simulink model "COSTEP_Auto"  (R2024b)
settings: Solver=FixedStepAuto  StartTime=0.0  StopTime=25  FixedStep=1/3600  RelTol=1e-3
model workspace (MAT data in the model file):
  AD : Simulink.Parameter (value not decoded)
  AG : Simulink.Parameter (value not decoded)
  AH : Simulink.Parameter (value not decoded)
  AV : Simulink.Parameter (value not decoded)
  AVP : Simulink.Parameter (value not decoded)
  BCHL : Simulink.Parameter (value not decoded)
  BCHV : Simulink.Parameter (value not decoded)
  BD : Simulink.Parameter (value not decoded)
  BG : Simulink.Parameter (value not decoded)
  BH : Simulink.Parameter (value not decoded)
  BVP : Simulink.Parameter (value not decoded)
  CD : Simulink.Parameter (value not decoded)
  CG : Simulink.Parameter (value not decoded)
  CH : Simulink.Parameter (value not decoded)
  CVP : Simulink.Parameter (value not decoded)
  ISV : Simulink.Parameter (value not decoded)
  XMW : Simulink.Parameter (value not decoded)
  XNS : Simulink.Parameter (value not decoded)
  XNS2 : Simulink.Parameter (value not decoded)
  XNS3 : Simulink.Parameter (value not decoded)
  XNSE : Simulink.Parameter (value not decoded)
values from neighbouring files (symbols this model uses):
  DD = SimData{4,1}{1,2}    [Auto_run_COSTEP.m]    (also in Run_COSTEP.m)
  G = SimData{2,1}(j,2)    [Auto_run_COSTEP.m]    (also in G.mat = [4243534565 7854912354 3456432354 1731738903 4346024432 5784; Run_COSTEP.m)
  IDV = SimData{3,1}(1:20,j)    [Auto_run_COSTEP.m]    (also in IDV.mat = [0 0 0 0 0 0 0 0 0 0 0 0 ... (812 elements, 28x29)]; Run_COSTEP.m = SimData{3,1}(1:28,j))
symbols that are objects in the model workspace (value not decoded): AD, AG, AH, AV, AVP, BD, BG, BH, BVP, CD, CG, CH, CVP, XMW, XNS, XNS2, XNS3, XNSE
undefined symbols (not defined in the file or in its folder): magnitude, msgbox, SETPT, XMEAS, XMV
libraries: mylib x304, dspindex x31
(part 5 of 13)

== system COSTEP_Auto/Process Measurements/Product analysis/Subsystem ==
  <XST(I;13)> : Inport
  Bus Selector : BusSelector  OutputSignals=XMNS(37),XMNS(38),XMNS(39),XMNS(40),XMNS(41)
  Process Noise I=37-{1..4,41} (5 alike) : mylib/Process Noise I=37-41  SystemSampleTime=-1  VariantActivationTime=update diagram  AllowFlexibleInterface=on  Latency=0  AutoFrameSizeCalculation=off
  Subsystem : Subsystem
  XMEAS(37) : Outport  VectorParamsAs1DForOutWhenUnconnected=off
  XMEAS(38) : Outport  Port=2  VectorParamsAs1DForOutWhenUnconnected=off
  XMEAS(39) : Outport  Port=3  VectorParamsAs1DForOutWhenUnconnected=off
  XMEAS(40) : Outport  Port=4  VectorParamsAs1DForOutWhenUnconnected=off
  XMEAS(41) : Outport  Port=5  VectorParamsAs1DForOutWhenUnconnected=off
  wires:
  Process Noise I=37-41/1 -> XMEAS(37)/1
  Bus Selector/1 -> Process Noise I=37-41/2  "<XMNS(37)>"
  Process Noise I=37-1/1 -> XMEAS(38)/1
  Bus Selector/2 -> Process Noise I=37-1/2  "<XMNS(38)>"
  Process Noise I=37-2/1 -> XMEAS(39)/1
  Bus Selector/3 -> Process Noise I=37-2/2  "<XMNS(39)>"
  Process Noise I=37-3/1 -> XMEAS(40)/1
  Bus Selector/4 -> Process Noise I=37-3/2  "<XMNS(40)>"
  Process Noise I=37-4/1 -> XMEAS(41)/1
  Bus Selector/5 -> Process Noise I=37-4/2  "<XMNS(41)>"
  <XST(I;13)>/1 -> Subsystem/1(XST)
  Subsystem/1("XCMP(37) ") -> Process Noise I=37-41/1
  Subsystem/2("XCMP(38) ") -> Process Noise I=37-1/1
  Subsystem/3("XCMP(39) ") -> Process Noise I=37-2/1
  Subsystem/4("XCMP(40) ") -> Process Noise I=37-3/1
  Subsystem/5("XCMP(41) ") -> Process Noise I=37-4/1
  [XMNS3] -> Bus Selector/1

== system COSTEP_Auto/Process Measurements/Purge gas analysis/Subsystem ==
  <XST(I;10)> : Inport
  Bus Selector : BusSelector  OutputSignals=XMNS(29),XMNS(30),XMNS(31),XMNS(32),XMNS(33),XMNS(34),XMNS(35),XMNS(36)
  Process Noise I=23-{1..7,36} (8 alike) : mylib/Process Noise I=23-36  SystemSampleTime=-1  VariantActivationTime=update diagram  AllowFlexibleInterface=on  Latency=0  AutoFrameSizeCalculation=off
  Subsystem : Subsystem
  XMEAS(29) : Outport  VectorParamsAs1DForOutWhenUnconnected=off
  XMEAS(30) : Outport  Port=2  VectorParamsAs1DForOutWhenUnconnected=off
  XMEAS(31) : Outport  Port=3  VectorParamsAs1DForOutWhenUnconnected=off
  XMEAS(32) : Outport  Port=4  VectorParamsAs1DForOutWhenUnconnected=off
  XMEAS(33) : Outport  Port=5  VectorParamsAs1DForOutWhenUnconnected=off
  XMEAS(34) : Outport  Port=6  VectorParamsAs1DForOutWhenUnconnected=off
  XMEAS(35) : Outport  Port=7  VectorParamsAs1DForOutWhenUnconnected=off
  XMEAS(36) : Outport  Port=8  VectorParamsAs1DForOutWhenUnconnected=off
  wires:
  Process Noise I=23-36/1 -> XMEAS(29)/1
  Process Noise I=23-1/1 -> XMEAS(30)/1
  Bus Selector/2 -> Process Noise I=23-1/2  "<XMNS(30)>"
  Process Noise I=23-2/1 -> XMEAS(31)/1
  Process Noise I=23-3/1 -> XMEAS(32)/1
  Process Noise I=23-4/1 -> XMEAS(33)/1
  Process Noise I=23-5/1 -> XMEAS(34)/1
  Process Noise I=23-6/1 -> XMEAS(35)/1
  Process Noise I=23-7/1 -> XMEAS(36)/1
  Bus Selector/7 -> Process Noise I=23-6/2  "<XMNS(35)>"
  Bus Selector/8 -> Process Noise I=23-7/2  "<XMNS(36)>"
  Bus Selector/6 -> Process Noise I=23-5/2  "<XMNS(34)>"
  Bus Selector/5 -> Process Noise I=23-4/2  "<XMNS(33)>"
  Bus Selector/4 -> Process Noise I=23-3/2  "<XMNS(32)>"
  Bus Selector/3 -> Process Noise I=23-2/2  "<XMNS(31)>"
  Bus Selector/1 -> Process Noise I=23-36/2  "<XMNS(29)>"
  <XST(I;10)>/1 -> Subsystem/1(XST)
  Subsystem/1("XCMP(29) ") -> Process Noise I=23-36/1
  Subsystem/2("XCMP(30) ") -> Process Noise I=23-1/1
  Subsystem/3("XCMP(31) ") -> Process Noise I=23-2/1
  Subsystem/4("XCMP(32) ") -> Process Noise I=23-3/1
  Subsystem/5("XCMP(33) ") -> Process Noise I=23-4/1
  Subsystem/6("XCMP(34) ") -> Process Noise I=23-5/1
  Subsystem/7("XCMP(35) ") -> Process Noise I=23-6/1
  Subsystem/8("XCMP(36) ") -> Process Noise I=23-7/1
  [XMNS2] -> Bus Selector/1

== system COSTEP_Auto/Process Measurements/Reactor feed analysis/Subsystem ==
  <XST(I;6) = XST(I;7)> : Inport
  Bus Selector : BusSelector  OutputSignals=XMNS(23),XMNS(24),XMNS(25),XMNS(26),XMNS(27),XMNS(28)
  Process Noise I=23-{1..5,36} (6 alike) : mylib/Process Noise I=23-36  SystemSampleTime=-1  VariantActivationTime=update diagram  AllowFlexibleInterface=on  Latency=0  AutoFrameSizeCalculation=off
  Subsystem : Subsystem
  XMEAS(23) : Outport  VectorParamsAs1DForOutWhenUnconnected=off
  XMEAS(24) : Outport  Port=2  VectorParamsAs1DForOutWhenUnconnected=off
  XMEAS(25) : Outport  Port=3  VectorParamsAs1DForOutWhenUnconnected=off
  XMEAS(26) : Outport  Port=4  VectorParamsAs1DForOutWhenUnconnected=off
  XMEAS(27) : Outport  Port=5  VectorParamsAs1DForOutWhenUnconnected=off
  XMEAS(28) : Outport  Port=6  VectorParamsAs1DForOutWhenUnconnected=off
  wires:
  Process Noise I=23-36/1 -> XMEAS(23)/1
  Bus Selector/1 -> Process Noise I=23-36/2  "<XMNS(23)>"
  Process Noise I=23-1/1 -> XMEAS(24)/1
  Process Noise I=23-2/1 -> XMEAS(25)/1
  Process Noise I=23-3/1 -> XMEAS(26)/1
  Process Noise I=23-4/1 -> XMEAS(27)/1
  Process Noise I=23-5/1 -> XMEAS(28)/1
  Bus Selector/2 -> Process Noise I=23-1/2  "<XMNS(24)>"
  Bus Selector/3 -> Process Noise I=23-2/2  "<XMNS(25)>"
  Bus Selector/4 -> Process Noise I=23-3/2  "<XMNS(26)>"
  Bus Selector/6 -> Process Noise I=23-5/2  "<XMNS(28)>"
  <XST(I;6) = XST(I;7)>/1 -> Subsystem/1(XST)
  Subsystem/1(XCMP(23)1) -> Process Noise I=23-36/1
  Subsystem/2(XCMP(24)1) -> Process Noise I=23-1/1
  Subsystem/3(XCMP(25)1) -> Process Noise I=23-2/1
  Subsystem/4(XCMP(26)1) -> Process Noise I=23-3/1
  Subsystem/5(XCMP(27)1) -> Process Noise I=23-4/1
  Subsystem/6(XCMP(28)1) -> Process Noise I=23-5/1
  [XMNS2] -> Bus Selector/1
  Bus Selector/5 -> Process Noise I=23-4/2  "<XMNS(27)>"

== system COSTEP_Auto/Process Measurements/Subsystem3/Reactor Feed  ==
  " " : Constant  Value=35.3145
  "  " : Constant  Value=0.359
  Add : Sum
  Bus Selector : BusSelector  OutputSignals=signal1.FTM(6) = FTM(7)
  Bus Selector1 : BusSelector  OutputSignals=XMNS(6)
  Product1 : Product  Inputs=**/
  "XMEAS(6) " : Outport  VectorParamsAs1DForOutWhenUnconnected=off
  wires:
  " "/1 -> Product1/3
  "  "/1 -> Product1/2
  [PropertiesStream6] -> Bus Selector/1
  Bus Selector/1 -> Product1/1  "<FTM(6) = FTM(7)>"
  Product1/1 -> Add/1
  Add/1 -> "XMEAS(6) "/1  "XMEAS(6)"
  Bus Selector1/1 -> Add/2  "<XMNS(6)>"
  [XMNS] -> Bus Selector1/1

== system COSTEP_Auto/Process Measurements/Subsystem3/Reactor Level ==
  " " : Sum  Inputs=+-
  "    " : Constant  Value=84.6
  "      " : Constant  Value=666.7
  "       " : Constant  Value=100
  Add : Sum
  Bus Selector1 : BusSelector  OutputSignals=XMNS(8)
  XMEAS(8) : Product  Inputs=*/*
  "XMEAS(8) " : Outport  VectorParamsAs1DForOutWhenUnconnected=off
  wires:
  " "/1 -> XMEAS(8)/1
  "       "/1 -> XMEAS(8)/3
  "    "/1 -> " "/2
  [VLR] -> " "/1
  "      "/1 -> XMEAS(8)/2
  XMEAS(8)/1 -> Add/1
  Add/1 -> "XMEAS(8) "/1  "XMEAS(8)"
  Bus Selector1/1 -> Add/2  "<XMNS(8)>"
  [XMNS] -> Bus Selector1/1

== system COSTEP_Auto/Process Measurements/Subsystem3/Reactor Pressure ==
  " " : Sum  Inputs=+-
  "    " : Constant  Value=760
  "       " : Constant  Value=101.325
  Add : Sum
  Bus Selector1 : BusSelector  OutputSignals=XMNS(7)
  XMEAS(7) : Product  Inputs=*/*
  "XMEAS(7) " : Outport  VectorParamsAs1DForOutWhenUnconnected=off
  wires:
  " "/1 -> XMEAS(7)/1
  "       "/1 -> XMEAS(7)/3
  "    "/1 -> XMEAS(7)/2, " "/2
  [PTR] -> " "/1
  XMEAS(7)/1 -> Add/1
  Add/1 -> "XMEAS(7) "/1  "XMEAS(7)"
  Bus Selector1/1 -> Add/2  "<XMNS(7)>"
  [XMNS] -> Bus Selector1/1

== system COSTEP_Auto/Process Measurements/Subsystem3/Reactor Temperature ==
  Add : Sum
  Bus Selector1 : BusSelector  OutputSignals=XMNS(9)
  "XMEAS(9) " : Outport  VectorParamsAs1DForOutWhenUnconnected=off
  wires:
  [TCR] -> Add/1
  Add/1 -> "XMEAS(9) "/1  "XMEAS(9)"
  Bus Selector1/1 -> Add/2  "<XMNS(9)>"
  [XMNS] -> Bus Selector1/1

== system COSTEP_Auto/Process Measurements/Subsystem4/Purge Rate ==
  " " : Constant  Value=35.3145
  "  " : Constant  Value=0.359
  Add : Sum
  Bus Selector : BusSelector  OutputSignals=signal1.FTM(10)
  Bus Selector1 : BusSelector  OutputSignals=XMNS(10)
  Product1 : Product  Inputs=**/
  "XMEAS(10) " : Outport  VectorParamsAs1DForOutWhenUnconnected=off
  wires:
  " "/1 -> Product1/3
  Bus Selector/1 -> Product1/1  "<FTM(10)>"
  "  "/1 -> Product1/2
  [PropertiesStream10] -> Bus Selector/1
  Product1/1 -> Add/1
  Add/1 -> "XMEAS(10) "/1  "XMEAS(10)"
  Bus Selector1/1 -> Add/2  "<XMNS(10)>"
  [XMNS] -> Bus Selector1/1

== system COSTEP_Auto/Process Measurements/Subsystem4/Separator Level ==
  " " : Sum  Inputs=+-
  "    " : Constant  Value=27.5
  "      " : Constant  Value=290
  "       " : Constant  Value=100
  Add : Sum
  Bus Selector1 : BusSelector  OutputSignals=XMNS(12)
  XMEAS(12) : Product  Inputs=*/*
  "XMEAS(12) " : Outport  VectorParamsAs1DForOutWhenUnconnected=off
  wires:
  " "/1 -> XMEAS(12)/1
  "       "/1 -> XMEAS(12)/3
  "    "/1 -> " "/2
  [VLS] -> " "/1
  "      "/1 -> XMEAS(12)/2
  XMEAS(12)/1 -> Add/1
  Add/1 -> "XMEAS(12) "/1  "XMEAS(12)"
  [XMNS] -> Bus Selector1/1
  Bus Selector1/1 -> Add/2  "<XMNS(12)>"

== system COSTEP_Auto/Process Measurements/Subsystem4/Separator Pressure ==
  "       1" : Constant  Value=101.325
  "    1" : Constant  Value=760
  " 1" : Sum  Inputs=+-
  Add : Sum
  Bus Selector1 : BusSelector  OutputSignals=XMNS(13)
  XMEAS(13) : Product  Inputs=*/*
  "XMEAS(13) " : Outport  VectorParamsAs1DForOutWhenUnconnected=off
  wires:
  "       1"/1 -> XMEAS(13)/3
  "    1"/1 -> XMEAS(13)/2, " 1"/2
  " 1"/1 -> XMEAS(13)/1
  [PTS] -> " 1"/1
  XMEAS(13)/1 -> Add/1
  Add/1 -> "XMEAS(13) "/1  "XMEAS(13)"
  [XMNS] -> Bus Selector1/1
  Bus Selector1/1 -> Add/2  "<XMNS(13)>"

== system COSTEP_Auto/Process Measurements/Subsystem4/Separator Temperature ==
  Add : Sum
  Bus Selector1 : BusSelector  OutputSignals=XMNS(11)
  "XMEAS(11) " : Outport  VectorParamsAs1DForOutWhenUnconnected=off
  wires:
  [TCS] -> Add/1
  Add/1 -> "XMEAS(11) "/1  "XMEAS(11)"
  [XMNS] -> Bus Selector1/1
  Bus Selector1/1 -> Add/2  "<XMNS(11)>"

== system COSTEP_Auto/Process Measurements/Subsystem4/Separator Underflow ==
  "       " : Constant  Value=35.3145
  Add : Sum
  Bus Selector : BusSelector  OutputSignals=signal1.FTM(11)
  Bus Selector1 : BusSelector  OutputSignals=XMNS(14)
  XMEAS(14) : Product  Inputs=*//
  "XMEAS(14) " : Outport  VectorParamsAs1DForOutWhenUnconnected=off
  wires:
  "       "/1 -> XMEAS(14)/3
  [DLS] -> XMEAS(14)/2
  [PropertiesStream11] -> Bus Selector/1
  Bus Selector/1 -> XMEAS(14)/1  "<FTM(11)>"
  XMEAS(14)/1 -> Add/1
  Add/1 -> "XMEAS(14) "/1  "XMEAS(14)"
  [XMNS] -> Bus Selector1/1
  Bus Selector1/1 -> Add/2  "<XMNS(14)>"

== system COSTEP_Auto/Process Measurements/Subsystem5/Stripper Level ==
  " " : Sum  Inputs=+-
  "    " : Constant  Value=78.25
  "       " : Constant  Value=100
  Add : Sum
  Bus Selector1 : BusSelector  OutputSignals=XMNS(15)
  VTC Total Volume of Stripper ft³ : Constant  Value=156.5
  XMEAS(15) : Product  Inputs=*/*
  "XMEAS(15) " : Outport  VectorParamsAs1DForOutWhenUnconnected=off
  wires:
  " "/1 -> XMEAS(15)/1
  "       "/1 -> XMEAS(15)/3
  "    "/1 -> " "/2
  [VLC] -> " "/1
  VTC Total Volume of Stripper ft³/1 -> XMEAS(15)/2
  XMEAS(15)/1 -> Add/1
  Add/1 -> "XMEAS(15) "/1  "XMEAS(15)"
  [XMNS] -> Bus Selector1/1
  Bus Selector1/1 -> Add/2  "<XMNS(15)>"

== system COSTEP_Auto/Process Measurements/Subsystem5/Stripper Pressure ==
  "    " : Constant  Value=760
  "         " : Constant  Value=101.325
  Add : Sum
  Bus Selector1 : BusSelector  OutputSignals=XMNS(16)
  Subtract : Sum  Inputs=+-
  XMEAS(16) : Product  Inputs=*/*
  "XMEAS(16) " : Outport  VectorParamsAs1DForOutWhenUnconnected=off
  wires:
  "    "/1 -> Subtract/2, XMEAS(16)/2
  [PTV] -> Subtract/1
  "         "/1 -> XMEAS(16)/3
  Subtract/1 -> XMEAS(16)/1
  XMEAS(16)/1 -> Add/1
  Add/1 -> "XMEAS(16) "/1  "XMEAS(16)"
  [XMNS] -> Bus Selector1/1
  Bus Selector1/1 -> Add/2  "<XMNS(16)>"

== system COSTEP_Auto/Process Measurements/Subsystem5/Stripper Steam Flow ==
  Add : Sum
  Bus Selector1 : BusSelector  OutputSignals=XMNS(19)
  Constant : Constant  Value=0.454
  Constant1 : Constant  Value=1.04E3
  XMEAS(19) : Product  Inputs=3
  "XMEAS(19) " : Outport  VectorParamsAs1DForOutWhenUnconnected=off
  wires:
  Constant1/1 -> XMEAS(19)/2
  [QUC] -> XMEAS(19)/1
  Constant/1 -> XMEAS(19)/3
  XMEAS(19)/1 -> Add/1
  Add/1 -> "XMEAS(19) "/1  "XMEAS(19)"
  [XMNS] -> Bus Selector1/1
  Bus Selector1/1 -> Add/2  "<XMNS(19)>"

== system COSTEP_Auto/Process Measurements/Subsystem5/Stripper Temperature ==
  Add : Sum
  Bus Selector1 : BusSelector  OutputSignals=XMNS(18)
  "XMEAS(18) " : Outport  VectorParamsAs1DForOutWhenUnconnected=off
  wires:
  [TCC] -> Add/1
  Add/1 -> "XMEAS(18) "/1  "XMEAS(18)"
  [XMNS] -> Bus Selector1/1
  Bus Selector1/1 -> Add/2  "<XMNS(18)>"

== system COSTEP_Auto/Process Measurements/Subsystem5/Stripper Underflow ==
  "       " : Constant  Value=35.3145
  Add : Sum
  Bus Selector : BusSelector  OutputSignals=FTM(13)
  Bus Selector1 : BusSelector  OutputSignals=XMNS(17)
  XMEAS(17) : Product  Inputs=*//
  "XMEAS(17) " : Outport  VectorParamsAs1DForOutWhenUnconnected=off
  wires:
  "       "/1 -> XMEAS(17)/3
  [DLC] -> XMEAS(17)/2
  [PropertiesStream13] -> Bus Selector/1
  Bus Selector/1 -> XMEAS(17)/1  "<FTM(13)>"
  XMEAS(17)/1 -> Add/1
  Add/1 -> "XMEAS(17) "/1  "XMEAS(17)"
  [XMNS] -> Bus Selector1/1
  Bus Selector1/1 -> Add/2  "<XMNS(17)>"

== system COSTEP_Auto/Random number generator/Disturbances I=1-9/Subsystem1 ==
  IDVWLK(2) : Inport
  G : Inport  Port=2
  DIST(2)_0 : Subsystem
  Disturbance calculations I=1-9 : mylib/Disturbance calculations I=1-9  SystemSampleTime=-1  VariantActivationTime=update diagram  AllowFlexibleInterface=on  Latency=0  AutoFrameSizeCalculation=off
  Subsystem : Subsystem
      mask Display: color('Blue'),disp('Disturbance constants')
  TESUB8 : mylib/TESUB8  SystemSampleTime=-1  VariantActivationTime=update diagram  AllowFlexibleInterface=on  Latency=0  AutoFrameSizeCalculation=off
  TESUB8(2,Time) : Outport  VectorParamsAs1DForOutWhenUnconnected=off
  G_NEW : Outport  Port=2  VectorParamsAs1DForOutWhenUnconnected=off
  wires:
  TESUB8/1 -> TESUB8(2,Time)/1
  Disturbance calculations I=1-9/1 -> TESUB8/1
  Disturbance calculations I=1-9/2 -> G_NEW/1
  IDVWLK(2)/1 -> Disturbance calculations I=1-9/1
  DIST(2)_0/1(DIST) -> Disturbance calculations I=1-9/4
  G/1 -> Disturbance calculations I=1-9/2
  Subsystem/1(Out1) -> Disturbance calculations I=1-9/3

== system COSTEP_Auto/Random number generator/Disturbances I=1-9/Subsystem10 ==
  IDVWLK(1) : Inport
  G : Inport  Port=2
  DIST(1)_0 : Subsystem
  Disturbance calculations I=1-9 : mylib/Disturbance calculations I=1-9  SystemSampleTime=-1  VariantActivationTime=update diagram  AllowFlexibleInterface=on  Latency=0  AutoFrameSizeCalculation=off
  Subsystem : Subsystem
      mask Display: color('Blue'),disp('Disturbance constants')
  TESUB8 : mylib/TESUB8  SystemSampleTime=-1  VariantActivationTime=update diagram  AllowFlexibleInterface=on  Latency=0  AutoFrameSizeCalculation=off
  TESUB8(1,Time) : Outport  VectorParamsAs1DForOutWhenUnconnected=off
  G_NEW : Outport  Port=2  VectorParamsAs1DForOutWhenUnconnected=off
  wires:
  TESUB8/1 -> TESUB8(1,Time)/1
  Disturbance calculations I=1-9/1 -> TESUB8/1
  Disturbance calculations I=1-9/2 -> G_NEW/1
  IDVWLK(1)/1 -> Disturbance calculations I=1-9/1
  DIST(1)_0/1(DIST) -> Disturbance calculations I=1-9/4
  G/1 -> Disturbance calculations I=1-9/2
  Subsystem/1(Out1) -> Disturbance calculations I=1-9/3

== system COSTEP_Auto/Random number generator/Disturbances I=1-9/Subsystem2 ==
  IDVWLK(3) : Inport
  G : Inport  Port=2
  DIST(3)_0 : Subsystem
  Disturbance calculations I=1-9 : mylib/Disturbance calculations I=1-9  SystemSampleTime=-1  VariantActivationTime=update diagram  AllowFlexibleInterface=on  Latency=0  AutoFrameSizeCalculation=off
  Subsystem : Subsystem
      mask Display: color('Blue'),disp('Disturbance constants')
  TESUB8 : mylib/TESUB8  SystemSampleTime=-1  VariantActivationTime=update diagram  AllowFlexibleInterface=on  Latency=0  AutoFrameSizeCalculation=off
  TESUB8(3,Time) : Outport  VectorParamsAs1DForOutWhenUnconnected=off
  G_NEW : Outport  Port=2  VectorParamsAs1DForOutWhenUnconnected=off
  wires:
  TESUB8/1 -> TESUB8(3,Time)/1
  Disturbance calculations I=1-9/1 -> TESUB8/1
  Disturbance calculations I=1-9/2 -> G_NEW/1
  IDVWLK(3)/1 -> Disturbance calculations I=1-9/1
  DIST(3)_0/1(DIST) -> Disturbance calculations I=1-9/4
  G/1 -> Disturbance calculations I=1-9/2
  Subsystem/1(Out1) -> Disturbance calculations I=1-9/3

== system COSTEP_Auto/Random number generator/Disturbances I=1-9/Subsystem3 ==
  IDVWLK(4) : Inport
  G : Inport  Port=2
  DIST(4)_0 : Subsystem
  Disturbance calculations I=1-9 : mylib/Disturbance calculations I=1-9  SystemSampleTime=-1  VariantActivationTime=update diagram  AllowFlexibleInterface=on  Latency=0  AutoFrameSizeCalculation=off
  Subsystem : Subsystem
      mask Display: color('Blue'),disp('Disturbance constants')
  TESUB8 : mylib/TESUB8  SystemSampleTime=-1  VariantActivationTime=update diagram  AllowFlexibleInterface=on  Latency=0  AutoFrameSizeCalculation=off
  TESUB8(4,Time) : Outport  VectorParamsAs1DForOutWhenUnconnected=off
  G_NEW : Outport  Port=2  VectorParamsAs1DForOutWhenUnconnected=off
  wires:
  TESUB8/1 -> TESUB8(4,Time)/1
  Disturbance calculations I=1-9/1 -> TESUB8/1
  Disturbance calculations I=1-9/2 -> G_NEW/1
  IDVWLK(4)/1 -> Disturbance calculations I=1-9/1
  DIST(4)_0/1(DIST) -> Disturbance calculations I=1-9/4
  G/1 -> Disturbance calculations I=1-9/2
  Subsystem/1(Out1) -> Disturbance calculations I=1-9/3

== system COSTEP_Auto/Random number generator/Disturbances I=1-9/Subsystem4 ==
  IDVWLK(5) : Inport
  G : Inport  Port=2
  DIST(5)_0 : Subsystem
  Disturbance calculations I=1-9 : mylib/Disturbance calculations I=1-9  SystemSampleTime=-1  VariantActivationTime=update diagram  AllowFlexibleInterface=on  Latency=0  AutoFrameSizeCalculation=off
  Subsystem : Subsystem
      mask Display: color('Blue'),disp('Disturbance constants')
  TESUB8 : mylib/TESUB8  SystemSampleTime=-1  VariantActivationTime=update diagram  AllowFlexibleInterface=on  Latency=0  AutoFrameSizeCalculation=off
  TESUB8(5,Time) : Outport  VectorParamsAs1DForOutWhenUnconnected=off
  G_NEW : Outport  Port=2  VectorParamsAs1DForOutWhenUnconnected=off
  wires:
  TESUB8/1 -> TESUB8(5,Time)/1
  Disturbance calculations I=1-9/1 -> TESUB8/1
  Disturbance calculations I=1-9/2 -> G_NEW/1
  IDVWLK(5)/1 -> Disturbance calculations I=1-9/1
  DIST(5)_0/1(DIST) -> Disturbance calculations I=1-9/4
  Subsystem/1(Out1) -> Disturbance calculations I=1-9/3
  G/1 -> Disturbance calculations I=1-9/2

== system COSTEP_Auto/Random number generator/Disturbances I=1-9/Subsystem5 ==
  IDVWLK(6) : Inport
  G : Inport  Port=2
  DIST(6)_0 : Subsystem
  Disturbance calculations I=1-9 : mylib/Disturbance calculations I=1-9  SystemSampleTime=-1  VariantActivationTime=update diagram  AllowFlexibleInterface=on  Latency=0  AutoFrameSizeCalculation=off
  Subsystem : Subsystem
      mask Display: color('Blue'),disp('Disturbance constants')
  TESUB8 : mylib/TESUB8  SystemSampleTime=-1  VariantActivationTime=update diagram  AllowFlexibleInterface=on  Latency=0  AutoFrameSizeCalculation=off
  TESUB8(6,Time) : Outport  VectorParamsAs1DForOutWhenUnconnected=off
  G_NEW : Outport  Port=2  VectorParamsAs1DForOutWhenUnconnected=off
  wires:
  TESUB8/1 -> TESUB8(6,Time)/1
  Disturbance calculations I=1-9/1 -> TESUB8/1
  Disturbance calculations I=1-9/2 -> G_NEW/1
  IDVWLK(6)/1 -> Disturbance calculations I=1-9/1
  DIST(6)_0/1(DIST) -> Disturbance calculations I=1-9/4
  G/1 -> Disturbance calculations I=1-9/2
  Subsystem/1(Out1) -> Disturbance calculations I=1-9/3

== system COSTEP_Auto/Random number generator/Disturbances I=1-9/Subsystem6 ==
  IDVWLK(7) : Inport
  G : Inport  Port=2
  DIST(7)_0 : Subsystem
  Disturbance calculations I=1-9 : mylib/Disturbance calculations I=1-9  SystemSampleTime=-1  VariantActivationTime=update diagram  AllowFlexibleInterface=on  Latency=0  AutoFrameSizeCalculation=off
  Subsystem : Subsystem
      mask Display: color('Blue'),disp('Disturbance constants')
  TESUB8 : mylib/TESUB8  SystemSampleTime=-1  VariantActivationTime=update diagram  AllowFlexibleInterface=on  Latency=0  AutoFrameSizeCalculation=off
  TESUB8(7,Time) : Outport  VectorParamsAs1DForOutWhenUnconnected=off
  G_NEW : Outport  Port=2  VectorParamsAs1DForOutWhenUnconnected=off
  wires:
  TESUB8/1 -> TESUB8(7,Time)/1
  Disturbance calculations I=1-9/1 -> TESUB8/1
  IDVWLK(7)/1 -> Disturbance calculations I=1-9/1
  G/1 -> Disturbance calculations I=1-9/2
  Subsystem/1(Out1) -> Disturbance calculations I=1-9/3
  DIST(7)_0/1(DIST) -> Disturbance calculations I=1-9/4
  Disturbance calculations I=1-9/2 -> G_NEW/1

== system COSTEP_Auto/Random number generator/Disturbances I=1-9/Subsystem7 ==
  IDVWLK(8) : Inport
  G : Inport  Port=2
  DIST(8)_0 : Subsystem
  Disturbance calculations I=1-9 : mylib/Disturbance calculations I=1-9  SystemSampleTime=-1  VariantActivationTime=update diagram  AllowFlexibleInterface=on  Latency=0  AutoFrameSizeCalculation=off
  Subsystem : Subsystem
      mask Display: color('Blue'),disp('Disturbance constants')
  TESUB8 : mylib/TESUB8  SystemSampleTime=-1  VariantActivationTime=update diagram  AllowFlexibleInterface=on  Latency=0  AutoFrameSizeCalculation=off
  TESUB8(8,Time) : Outport  VectorParamsAs1DForOutWhenUnconnected=off
  G_NEW : Outport  Port=2  VectorParamsAs1DForOutWhenUnconnected=off
  wires:
  TESUB8/1 -> TESUB8(8,Time)/1
  Disturbance calculations I=1-9/1 -> TESUB8/1
  Disturbance calculations I=1-9/2 -> G_NEW/1
  IDVWLK(8)/1 -> Disturbance calculations I=1-9/1
  G/1 -> Disturbance calculations I=1-9/2
  Subsystem/1(Out1) -> Disturbance calculations I=1-9/3
  DIST(8)_0/1(DIST) -> Disturbance calculations I=1-9/4

== system COSTEP_Auto/Random number generator/Disturbances I=1-9/Subsystem8 ==
  IDVWLK(9) : Inport
  G : Inport  Port=2
  DIST(9)_0 : Subsystem
  Disturbance calculations I=1-9 : mylib/Disturbance calculations I=1-9  SystemSampleTime=-1  VariantActivationTime=update diagram  AllowFlexibleInterface=on  Latency=0  AutoFrameSizeCalculation=off
  Subsystem : Subsystem
      mask Display: color('Blue'),disp('Disturbance constants')
  TESUB8 : mylib/TESUB8  SystemSampleTime=-1  VariantActivationTime=update diagram  AllowFlexibleInterface=on  Latency=0  AutoFrameSizeCalculation=off
  TESUB8(9,Time) : Outport  VectorParamsAs1DForOutWhenUnconnected=off
  G_NEW : Outport  Port=2  VectorParamsAs1DForOutWhenUnconnected=off
  wires:
  TESUB8/1 -> TESUB8(9,Time)/1
  Disturbance calculations I=1-9/1 -> TESUB8/1
  Disturbance calculations I=1-9/2 -> G_NEW/1
  IDVWLK(9)/1 -> Disturbance calculations I=1-9/1
  G/1 -> Disturbance calculations I=1-9/2
  Subsystem/1(Out1) -> Disturbance calculations I=1-9/3
  DIST(9)_0/1(DIST) -> Disturbance calculations I=1-9/4

== system COSTEP_Auto/Random number generator/Disturbances I=10-12/Subsystem1 ==
  IDVWLK(11) : Inport
  G : Inport  Port=2
  DIST(11)_0 : Subsystem
  Subsystem2 : Subsystem
      mask Display: color('Blue'),disp('Disturbance constants')
  Subsystem3 : mylib/Subsystem3  SystemSampleTime=-1  VariantActivationTime=update diagram  AllowFlexibleInterface=on  Latency=0  AutoFrameSizeCalculation=off
  TESUB8 : mylib/TESUB8  SystemSampleTime=-1  VariantActivationTime=update diagram  AllowFlexibleInterface=on  Latency=0  AutoFrameSizeCalculation=off
  TESUB8(11,Time) : Outport  VectorParamsAs1DForOutWhenUnconnected=off
  G_NEW : Outport  Port=2  VectorParamsAs1DForOutWhenUnconnected=off
  wires:
  TESUB8/1 -> TESUB8(11,Time)/1
  Subsystem3/1 -> TESUB8/1
  IDVWLK(11)/1 -> Subsystem3/1
  G/1 -> Subsystem3/2
  Subsystem3/2 -> G_NEW/1
  Subsystem2/1(Out1) -> Subsystem3/3
  DIST(11)_0/1(DIST_0) -> Subsystem3/4

== system COSTEP_Auto/Random number generator/Disturbances I=10-12/Subsystem10 ==
  IDVWLK(10) : Inport
  G : Inport  Port=2
  DIST(10)_0 : Subsystem
  Subsystem2 : Subsystem
      mask Display: color('Blue'),disp('Disturbance constants')
  Subsystem3 : mylib/Subsystem3  SystemSampleTime=-1  VariantActivationTime=update diagram  AllowFlexibleInterface=on  Latency=0  AutoFrameSizeCalculation=off
  TESUB8 : mylib/TESUB8  SystemSampleTime=-1  VariantActivationTime=update diagram  AllowFlexibleInterface=on  Latency=0  AutoFrameSizeCalculation=off
  TESUB8(10,Time) : Outport  VectorParamsAs1DForOutWhenUnconnected=off
  G_NEW : Outport  Port=2  VectorParamsAs1DForOutWhenUnconnected=off
  wires:
  TESUB8/1 -> TESUB8(10,Time)/1
  Subsystem3/1 -> TESUB8/1
  IDVWLK(10)/1 -> Subsystem3/1
  G/1 -> Subsystem3/2
  Subsystem3/2 -> G_NEW/1
  Subsystem2/1(Out1) -> Subsystem3/3
  DIST(10)_0/1(DIST_0) -> Subsystem3/4

== system COSTEP_Auto/Random number generator/Disturbances I=10-12/Subsystem2 ==
  IDVWLK(12) : Inport
  G : Inport  Port=2
  DIST(12)_0 : Subsystem
  Subsystem2 : Subsystem
      mask Display: color('Blue'),disp('Disturbance constants')
  Subsystem3 : mylib/Subsystem3  SystemSampleTime=-1  VariantActivationTime=update diagram  AllowFlexibleInterface=on  Latency=0  AutoFrameSizeCalculation=off
  TESUB8 : mylib/TESUB8  SystemSampleTime=-1  VariantActivationTime=update diagram  AllowFlexibleInterface=on  Latency=0  AutoFrameSizeCalculation=off
  TESUB8(12,Time) : Outport  VectorParamsAs1DForOutWhenUnconnected=off
  G_NEW : Outport  Port=2  VectorParamsAs1DForOutWhenUnconnected=off
  wires:
  TESUB8/1 -> TESUB8(12,Time)/1
  Subsystem3/1 -> TESUB8/1
  IDVWLK(12)/1 -> Subsystem3/1
  G/1 -> Subsystem3/2
  Subsystem3/2 -> G_NEW/1
  Subsystem2/1(Out1) -> Subsystem3/3
  DIST(12)_0/1(DIST_0) -> Subsystem3/4

== system COSTEP_Auto/Random number generator/Process Measurements XMEAS(I) I=1-22/Subsystem ==
  XMNS : Inport
  Bus Creator : BusCreator  Inputs=22
  Demux : Demux  Outputs=22
  "XMNS " : Outport
  wires:
  XMNS/1 -> Demux/1
  Demux/1 -> Bus Creator/1  "XMNS(1)"
  Demux/2 -> Bus Creator/2  "XMNS(2)"
  Demux/3 -> Bus Creator/3  "XMNS(3)"
  Demux/4 -> Bus Creator/4  "XMNS(4)"
  Demux/5 -> Bus Creator/5  "XMNS(5)"
  Demux/6 -> Bus Creator/6  "XMNS(6)"
  Demux/7 -> Bus Creator/7  "XMNS(7)"
  Demux/8 -> Bus Creator/8  "XMNS(8)"
  Demux/9 -> Bus Creator/9  "XMNS(9)"
  Demux/10 -> Bus Creator/10  "XMNS(10)"
  Demux/11 -> Bus Creator/11  "XMNS(11)"
  Demux/12 -> Bus Creator/12  "XMNS(12)"
  Demux/13 -> Bus Creator/13  "XMNS(13)"
  Demux/14 -> Bus Creator/14  "XMNS(14)"
  Demux/15 -> Bus Creator/15  "XMNS(15)"
  Demux/16 -> Bus Creator/16  "XMNS(16)"
  Demux/17 -> Bus Creator/17  "XMNS(17)"
  Demux/18 -> Bus Creator/18  "XMNS(18)"
  Demux/19 -> Bus Creator/19  "XMNS(19)"
  Demux/20 -> Bus Creator/20  "XMNS(20)"
  Demux/21 -> Bus Creator/21  "XMNS(21)"
  Demux/22 -> Bus Creator/22  "XMNS(22)"
  Bus Creator/1 -> "XMNS "/1

== system COSTEP_Auto/Random number generator/Process Measurements XMEAS(I) I=23-36/Subsystem ==
  XMNS : Inport
  Bus Creator : BusCreator  Inputs=14
  Demux : Demux  Outputs=14
  "XMNS " : Outport
  wires:
  XMNS/1 -> Demux/1
  Demux/1 -> Bus Creator/1  "XMNS(23)"
  Demux/2 -> Bus Creator/2  "XMNS(24)"
  Demux/3 -> Bus Creator/3  "XMNS(25)"
  Demux/4 -> Bus Creator/4  "XMNS(26)"
  Demux/5 -> Bus Creator/5  "XMNS(27)"
  Demux/6 -> Bus Creator/6  "XMNS(28)"
  Demux/7 -> Bus Creator/7  "XMNS(29)"
  Demux/8 -> Bus Creator/8  "XMNS(30)"
  Demux/9 -> Bus Creator/9  "XMNS(31)"
  Demux/10 -> Bus Creator/10  "XMNS(32)"
  Demux/11 -> Bus Creator/11  "XMNS(33)"
  Demux/12 -> Bus Creator/12  "XMNS(34)"
  Demux/13 -> Bus Creator/13  "XMNS(35)"
  Demux/14 -> Bus Creator/14  "XMNS(36)"
  Bus Creator/1 -> "XMNS "/1

== system COSTEP_Auto/Random number generator/Process Measurements XMEAS(I) I=37-41/Subsystem ==
  XMNS : Inport
  Bus Creator : BusCreator  Inputs=5
  Demux : Demux  Outputs=5
  "XMNS " : Outport
  wires:
  XMNS/1 -> Demux/1
  Demux/1 -> Bus Creator/1  "XMNS(37)"
  Demux/2 -> Bus Creator/2  "XMNS(38)"
  Demux/3 -> Bus Creator/3  "XMNS(39)"
  Demux/4 -> Bus Creator/4  "XMNS(40)"
  Demux/5 -> Bus Creator/5  "XMNS(41)"
  Bus Creator/1 -> "XMNS "/1

== system COSTEP_Auto/Random number generator/Stream Measurements SMEAS/Subsystem ==
  XMNSE : Inport
  Bus Creator : BusCreator  Inputs=24
  Demux : Demux  Outputs=24
  "XMNSE " : Outport
  wires:
  XMNSE/1 -> Demux/1
  Demux/1 -> Bus Creator/1  "XMNSE(1)"
  Demux/2 -> Bus Creator/2  "XMNSE(2)"
  Demux/3 -> Bus Creator/3  "XMNSE(3)"
  Demux/4 -> Bus Creator/4  "XMNSE(4)"
  Demux/5 -> Bus Creator/5  "XMNSE(5)"
  Demux/6 -> Bus Creator/6  "XMNSE(6)"
  Demux/7 -> Bus Creator/7  "XMNSE(7)"
  Demux/8 -> Bus Creator/8  "XMNSE(8)"
  Demux/9 -> Bus Creator/9  "XMNSE(9)"
  Demux/10 -> Bus Creator/10  "XMNSE(10)"
  Demux/11 -> Bus Creator/11  "XMNSE(11)"
  Demux/12 -> Bus Creator/12  "XMNSE(12)"
  Demux/13 -> Bus Creator/13  "XMNSE(13)"
  Demux/14 -> Bus Creator/14  "XMNSE(14)"
  Demux/15 -> Bus Creator/15  "XMNSE(15)"
  Demux/16 -> Bus Creator/16  "XMNSE(16)"
  Demux/17 -> Bus Creator/17  "XMNSE(17)"
  Demux/18 -> Bus Creator/18  "XMNSE(18)"
  Demux/19 -> Bus Creator/19  "XMNSE(19)"
  Demux/20 -> Bus Creator/20  "XMNSE(20)"
  Demux/21 -> Bus Creator/21  "XMNSE(21)"
  Demux/22 -> Bus Creator/22  "XMNSE(22)"
  Bus Creator/1 -> "XMNSE "/1
  Demux/23 -> Bus Creator/23  "XMNSE(23)"
  Demux/24 -> Bus Creator/24  "XMNSE(24)"

== system COSTEP_Auto/Random number generator/Stream Measurements SMEAS Gas analysis/Gas Analysis Delay ==
  Clock : Clock
  Constant : Constant  Value=3600
  If : If  NumInputs=2  IfExpression=u1 > 0 & u2 == 0  ShowElse=off
  Math Function : Math  Operator=mod  SignedPower=on
  Merge : Merge
  Product : Product
  Subsystem : Subsystem
      mask Display: color('Blue'), disp('MOD\nFix');
  TGAS Delay 0.1h : Constant  Value=360
  IF(TGAS) : Outport  VectorParamsAs1DForOutWhenUnconnected=off
  wires:
  Product/1 -> Math Function/1
  TGAS Delay 0.1h/1 -> Subsystem/2(In2), Math Function/2
  Clock/1 -> Product/1, If/1
  If/1 -> IF(TGAS)/1
  Constant/1 -> Product/2
  Math Function/1 -> Subsystem/1(In1)
  Subsystem/2(Out2) -> Merge/2
  Subsystem/1(Out1) -> Merge/1
  Merge/1 -> If/2

== system COSTEP_Auto/Random number generator/Stream Measurements SMEAS Gas analysis/If Action Subsystem3 ==
  GE2 : Inport
  Action Port : ActionPort  ActionPortLabel=if(u1 > 0 & u2 == 0)
  Subsystem : Subsystem
  XMNS : Outport  OutputWhenDisabled=reset  InitialOutput=[0]  VectorParamsAs1DForOutWhenUnconnected=off
  GE3 : Outport  Port=2  OutputWhenDisabled=reset  InitialOutput=[0]  VectorParamsAs1DForOutWhenUnconnected=off
  wires:
  GE2/1 -> Subsystem/1(G)
  Subsystem/2(G_NEW) -> GE3/1
  Subsystem/1(XMNSE2) -> XMNS/1

== system COSTEP_Auto/Random number generator/Stream Measurements SMEAS Gas analysis/Subsystem ==
  In2 : Inport
  GE2 : Inport  Port=2
  If Action Subsystem : Subsystem  TreatAsAtomicUnit=on
  If Action Subsystem1 : Subsystem  TreatAsAtomicUnit=on
  If5 : If  IfExpression=u1 == 0
  Merge : Merge
  GE3 : Outport  VectorParamsAs1DForOutWhenUnconnected=off
  wires:
  In2/1 -> If Action Subsystem1/1(In1), If5/1
  If5/2 -> If Action Subsystem1/Action
  If Action Subsystem1/1(Out1) -> Merge/1
  If5/1 -> If Action Subsystem/Action
  If Action Subsystem/1(Out1) -> Merge/2
  GE2/1 -> If Action Subsystem/1(In1)
  Merge/1 -> GE3/1

== system COSTEP_Auto/Random number generator/Stream Measurements SMEAS Product analysis/Gas Analysis Delay ==
  Clock : Clock
  Constant : Constant  Value=3600
  If : If  NumInputs=2  IfExpression=u1 > 0 & u2 == 0  ShowElse=off
  Math Function : Math  Operator=mod  SignedPower=on
  Merge : Merge
  Product : Product
  Subsystem : Subsystem
      mask Display: color('Blue'), disp('MOD\nFix');
  TPROD Delay 0.25h : Constant  Value=900
  IF(TPROD) : Outport  VectorParamsAs1DForOutWhenUnconnected=off
  wires:
  Product/1 -> Math Function/1
  TPROD Delay 0.25h/1 -> Subsystem/2(In2), Math Function/2
  Clock/1 -> Product/1, If/1
  If/1 -> IF(TPROD)/1
  Constant/1 -> Product/2
  Math Function/1 -> Subsystem/1(In1)
  Subsystem/1(Out1) -> Merge/1
  Subsystem/2(Out2) -> Merge/2
  Merge/1 -> If/2

== system COSTEP_Auto/Random number generator/Stream Measurements SMEAS Product analysis/If Action Subsystem3 ==
  GE3 : Inport
  Action Port : ActionPort  ActionPortLabel=if(u1 > 0 & u2 == 0)
  Subsystem : Subsystem
  XMNSE : Outport  OutputWhenDisabled=reset  InitialOutput=[0]  VectorParamsAs1DForOutWhenUnconnected=off
  GE4 : Outport  Port=2  OutputWhenDisabled=reset  InitialOutput=[0]  VectorParamsAs1DForOutWhenUnconnected=off
  wires:
  GE3/1 -> Subsystem/1(G)
  Subsystem/2(G_NEW) -> GE4/1
  Subsystem/1(XMNSE3) -> XMNSE/1

== system COSTEP_Auto/Random number generator/Stream Measurements SMEAS Product analysis/Subsystem ==
  In2 : Inport
  GE3 : Inport  Port=2
  If Action Subsystem : Subsystem  TreatAsAtomicUnit=on
  If Action Subsystem1 : Subsystem  TreatAsAtomicUnit=on
  If5 : If  IfExpression=u1 == 0
  Merge : Merge
  GE4 : Outport  VectorParamsAs1DForOutWhenUnconnected=off
  wires:
  In2/1 -> If Action Subsystem1/1(In1), If5/1
  If5/2 -> If Action Subsystem1/Action
  If Action Subsystem1/1(Out1) -> Merge/1
  If5/1 -> If Action Subsystem/Action
  If Action Subsystem/1(Out1) -> Merge/2
  GE3/1 -> If Action Subsystem/1(In1)
  Merge/1 -> GE4/1

== system COSTEP_Auto/Reactor/Holdup of Components in Reactor/Holdup of Liquid Components in Reactor ==
  YY(1:8) : Inport  PortDimensions=8
  Bus Creator : BusCreator  Inputs=8
  Bus Selector : BusSelector  OutputSignals=YY(4),YY(5),YY(6),YY(7),YY(8)
  UCLR(1) Holdup of Component A (Liquid) in Reactor lb-mol : Constant  Value=0
  UCLR(2) Holdup of Component B (Liquid) in Reactor lb-mol : Constant  Value=0
  UCLR(3) Holdup of Component C (Liquid) in Reactor lb-mol : Constant  Value=0
  UCLR(4) Holdup of Component D (Liquid) in Reactor lb-mol : Gain
  UCLR(5) Holdup of Component E (Liquid) in Reactor lb-mol : Gain
  UCLR(6) Holdup of Component F (Liquid) in Reactor lb-mol : Gain
  UCLR(7) Holdup of Component G (Liquid) in Reactor lb-mol : Gain
  UCLR(8) Holdup of Component H (Liquid) in Reactor lb-mol : Gain
  UCLR : Outport  PortDimensions=8  VectorParamsAs1DForOutWhenUnconnected=off
  wires:
  UCLR(8) Holdup of Component H (Liquid) in Reactor lb-mol/1 -> Bus Creator/8  "UCLR(8)"
  UCLR(4) Holdup of Component D (Liquid) in Reactor lb-mol/1 -> Bus Creator/4  "UCLR(4)"
  UCLR(3) Holdup of Component C (Liquid) in Reactor lb-mol/1 -> Bus Creator/3  "UCLR(3)"
  UCLR(2) Holdup of Component B (Liquid) in Reactor lb-mol/1 -> Bus Creator/2  "UCLR(2)"
  UCLR(6) Holdup of Component F (Liquid) in Reactor lb-mol/1 -> Bus Creator/6  "UCLR(6)"
  UCLR(5) Holdup of Component E (Liquid) in Reactor lb-mol/1 -> Bus Creator/5  "UCLR(5)"
  UCLR(7) Holdup of Component G (Liquid) in Reactor lb-mol/1 -> Bus Creator/7  "UCLR(7)"
  UCLR(1) Holdup of Component A (Liquid) in Reactor lb-mol/1 -> Bus Creator/1  "UCLR(1)"
  Bus Selector/4 -> UCLR(7) Holdup of Component G (Liquid) in Reactor lb-mol/1  "<YY(7)>"
  Bus Selector/2 -> UCLR(5) Holdup of Component E (Liquid) in Reactor lb-mol/1  "<YY(5)>"
  Bus Selector/5 -> UCLR(8) Holdup of Component H (Liquid) in Reactor lb-mol/1  "<YY(8)>"
  Bus Selector/3 -> UCLR(6) Holdup of Component F (Liquid) in Reactor lb-mol/1  "<YY(6)>"
  YY(1:8)/1 -> Bus Selector/1
  Bus Selector/1 -> UCLR(4) Holdup of Component D (Liquid) in Reactor lb-mol/1  "<YY(4)>"
  Bus Creator/1 -> UCLR/1

== system COSTEP_Auto/Reactor/Holdup of Components in Reactor/Holdup of Vapour Components in Reactor ==
  YY(1:8) : Inport
  Bus Creator : BusCreator  Inputs=3
  Bus Selector : BusSelector  OutputSignals=YY(1),YY(2),YY(3)
  UCVR(1) Holdup of Component A (Vapour) in Reactor lb-mol : Gain
  UCVR(2) Holdup of Component B (Vapour) in Reactor lb-mol : Gain
  UCVR(3) Holdup of Component C (Vapour) in Reactor lb-mol : Gain
  UCVR : Outport  PortDimensions=3  VectorParamsAs1DForOutWhenUnconnected=off
  wires:
  UCVR(2) Holdup of Component B (Vapour) in Reactor lb-mol/1 -> Bus Creator/2  "UCVR(2)"
  Bus Selector/2 -> UCVR(2) Holdup of Component B (Vapour) in Reactor lb-mol/1  "<YY(2)>"
  Bus Selector/3 -> UCVR(3) Holdup of Component C (Vapour) in Reactor lb-mol/1  "<YY(3)>"
  UCVR(3) Holdup of Component C (Vapour) in Reactor lb-mol/1 -> Bus Creator/3  "UCVR(3)"
  UCVR(1) Holdup of Component A (Vapour) in Reactor lb-mol/1 -> Bus Creator/1  "UCVR(1)"
  Bus Creator/1 -> UCVR/1
  YY(1:8)/1 -> Bus Selector/1
  Bus Selector/1 -> UCVR(1) Holdup of Component A (Vapour) in Reactor lb-mol/1  "<YY(1)>"

== system COSTEP_Auto/Reactor/Holdup of Components in Reactor/Liquid Component Fraction in Reactor lb-mol ==
  UTLR : Inport
  UCLR : Inport  Port=2
  Bus Creator : BusCreator  Inputs=8
  Bus Selector : BusSelector  OutputSignals=UCLR(1),UCLR(2),UCLR(3),UCLR(4),UCLR(5),UCLR(6),UCLR(7),UCLR(8)
  XLR(1) : Product  Inputs=*/
  XLR(2) : Product  Inputs=*/
  XLR(3) : Product  Inputs=*/
  XLR(4) : Product  Inputs=*/
  XLR(5) : Product  Inputs=*/
  XLR(6) : Product  Inputs=*/
  XLR(7) : Product  Inputs=*/
  XLR(8) : Product  Inputs=*/
  XLR : Outport  VectorParamsAs1DForOutWhenUnconnected=off
  wires:
  XLR(5)/1 -> Bus Creator/5  "XLR(5)"
  Bus Selector/3 -> XLR(3)/1  "<UCLR(3)>"
  UTLR/1 -> XLR(8)/2, XLR(7)/2, XLR(6)/2, XLR(5)/2, XLR(4)/2, XLR(3)/2, XLR(2)/2, XLR(1)/2
  Bus Selector/7 -> XLR(7)/1  "<UCLR(7)>"
  XLR(8)/1 -> Bus Creator/8  "XLR(8)"
  XLR(7)/1 -> Bus Creator/7  "XLR(7)"
  Bus Selector/8 -> XLR(8)/1  "<UCLR(8)>"
  Bus Selector/5 -> XLR(5)/1  "<UCLR(5)>"
  Bus Selector/4 -> XLR(4)/1  "<UCLR(4)>"
  XLR(2)/1 -> Bus Creator/2  "XLR(2)"
  Bus Selector/6 -> XLR(6)/1  "<UCLR(6)>"
  XLR(3)/1 -> Bus Creator/3  "XLR(3)"
  UCLR/1 -> Bus Selector/1
  Bus Selector/1 -> XLR(1)/1  "<UCLR(1)>"
  XLR(4)/1 -> Bus Creator/4  "XLR(4)"
  Bus Selector/2 -> XLR(2)/1  "<UCLR(2)>"
  XLR(6)/1 -> Bus Creator/6  "XLR(6)"
  XLR(1)/1 -> Bus Creator/1  "XLR(1)"
  Bus Creator/1 -> XLR/1

== system COSTEP_Auto/Reactor/Holdup of Components in Reactor/Subsystem ==
  Properties of Stream 6 : Inport
  Bus Creator1 : BusCreator  Inputs=8
  Bus Selector1 : BusSelector  OutputSignals=FCM(I;6) = FCM(I;7)
  Multiport Selector : dspindex/Multiport Selector  rowsOrCols=Rows  idxCellArray={ 1,2,3,4,5,6,7,8}  idxErrMode=Clip Index
  FCM(I;7) : Outport  VectorParamsAs1DForOutWhenUnconnected=off
  wires:
  Multiport Selector/8 -> Bus Creator1/8  "FCM(8;7)"
  Multiport Selector/4 -> Bus Creator1/4  "FCM(4;7)"
  Multiport Selector/1 -> Bus Creator1/1  "FCM(1;7)"
  Bus Selector1/1 -> Multiport Selector/1  "<FCM(I;6) = FCM(I;7)>"
  Multiport Selector/6 -> Bus Creator1/6  "FCM(6;7)"
  Multiport Selector/2 -> Bus Creator1/2  "FCM(2;7)"
  Properties of Stream 6/1 -> Bus Selector1/1
  Multiport Selector/7 -> Bus Creator1/7  "FCM(7;7)"
  Multiport Selector/5 -> Bus Creator1/5  "FCM(5;7)"
  Multiport Selector/3 -> Bus Creator1/3  "FCM(3;7)"
  Bus Creator1/1 -> FCM(I;7)/1

== system COSTEP_Auto/Reactor/Holdup of Components in Reactor/Subsystem1 ==
  Bus Creator1 : BusCreator  Inputs=8
  Bus Selector2 : BusSelector  OutputSignals=signal1.FCM(I;8)
  Multiport Selector1 : dspindex/Multiport Selector  rowsOrCols=Rows  idxCellArray={ 1,2,3,4,5,6,7,8}  idxErrMode=Clip Index
  FCM(I;8) : Outport  VectorParamsAs1DForOutWhenUnconnected=off
  wires:
  Multiport Selector1/4 -> Bus Creator1/4  "FCM(4;8)"
  Multiport Selector1/5 -> Bus Creator1/5  "FCM(5;8)"
  Multiport Selector1/6 -> Bus Creator1/6  "FCM(6;8)"
  Multiport Selector1/3 -> Bus Creator1/3  "FCM(3;8)"
  Multiport Selector1/8 -> Bus Creator1/8  "FCM(8;8)"
  Bus Selector2/1 -> Multiport Selector1/1  "<FCM(I;8)>"
  Multiport Selector1/2 -> Bus Creator1/2  "FCM(2;8)"
  Multiport Selector1/7 -> Bus Creator1/7  "FCM(7;8)"
  Multiport Selector1/1 -> Bus Creator1/1  "FCM(1;8)"
  Bus Creator1/1 -> FCM(I;8)/1
  [PropertiesStream8] -> Bus Selector2/1

== system COSTEP_Auto/Reactor/Holdup of Components in Reactor/YP(1) ==
  FCM(1,7) : Inport
  CRXR(1) : Inport  Port=2
  FCM(1,8) : Inport  Port=3
  " YP(1)" : Sum  Inputs=+-+
  Bus Selector : BusSelector  OutputSignals=FCM(1;7)
  Bus Selector1 : BusSelector  OutputSignals=FCM(1;8)
  Bus Selector2 : BusSelector  OutputSignals=CRXR(1)
  Integration : mylib/Integration  SystemSampleTime=-1  VariantActivationTime=update diagram  AllowFlexibleInterface=on  Latency=0  AutoFrameSizeCalculation=off
  "YY(1) " : Constant  Value=10.40491389
  YY(1) : Outport  VectorParamsAs1DForOutWhenUnconnected=off
  wires:
  FCM(1,7)/1 -> Bus Selector/1
  Bus Selector/1 -> " YP(1)"/1  "<FCM(1;7)>"
  FCM(1,8)/1 -> Bus Selector1/1
  Bus Selector1/1 -> " YP(1)"/2  "<FCM(1;8)>"
  CRXR(1)/1 -> Bus Selector2/1
  Bus Selector2/1 -> " YP(1)"/3  "<CRXR(1)>"
  " YP(1)"/1 -> Integration/1
  "YY(1) "/1 -> Integration/2
  Integration/1 -> YY(1)/1

== system COSTEP_Auto/Reactor/Holdup of Components in Reactor/YP(2) ==
  FCM(2,7) : Inport
  FCM(2,8) : Inport  Port=2
  Bus Selector : BusSelector  OutputSignals=FCM(2;7)
  Bus Selector1 : BusSelector  OutputSignals=FCM(2;8)
  Integration : mylib/Integration  SystemSampleTime=-1  VariantActivationTime=update diagram  AllowFlexibleInterface=on  Latency=0  AutoFrameSizeCalculation=off
  "YP(2) " : Sum  Inputs=+-
  "YY(2) " : Constant  Value=4.363996017
  YY(2) : Outport  VectorParamsAs1DForOutWhenUnconnected=off
  wires:
  FCM(2,8)/1 -> Bus Selector1/1
  FCM(2,7)/1 -> Bus Selector/1
  Bus Selector/1 -> "YP(2) "/1  "<FCM(2;7)>"
  Bus Selector1/1 -> "YP(2) "/2  "<FCM(2;8)>"
  "YP(2) "/1 -> Integration/1
  "YY(2) "/1 -> Integration/2
  Integration/1 -> YY(2)/1

== system COSTEP_Auto/Reactor/Holdup of Components in Reactor/YP(3) ==
  FCM(3,7) : Inport
  CRXR(3) : Inport  Port=2
  FCM(3,8) : Inport  Port=3
  " YP(3)" : Sum  Inputs=+-+
  Bus Selector : BusSelector  OutputSignals=CRXR(3)
  Bus Selector1 : BusSelector  OutputSignals=FCM(3;8)
  Bus Selector2 : BusSelector  OutputSignals=FCM(3;7)
  Integration : mylib/Integration  SystemSampleTime=-1  VariantActivationTime=update diagram  AllowFlexibleInterface=on  Latency=0  AutoFrameSizeCalculation=off
  "YY(3) " : Constant  Value=7.5700579737
  YY(3) : Outport  VectorParamsAs1DForOutWhenUnconnected=off
  wires:
  CRXR(3)/1 -> Bus Selector/1
  FCM(3,8)/1 -> Bus Selector1/1
  FCM(3,7)/1 -> Bus Selector2/1
  Bus Selector/1 -> " YP(3)"/3  "<CRXR(3)>"
  Bus Selector1/1 -> " YP(3)"/2  "<FCM(3;8)>"
  Bus Selector2/1 -> " YP(3)"/1  "<FCM(3;7)>"
  " YP(3)"/1 -> Integration/1
  "YY(3) "/1 -> Integration/2
  Integration/1 -> YY(3)/1

== system COSTEP_Auto/Reactor/Holdup of Components in Reactor/YP(4) ==
  FCM(4,7) : Inport
  CRXR(4) : Inport  Port=2
  FCM(4,8) : Inport  Port=3
  " " : Sum  Inputs=+-+
  Bus Selector : BusSelector  OutputSignals=CRXR(4)
  Bus Selector1 : BusSelector  OutputSignals=FCM(4;8)
  Bus Selector2 : BusSelector  OutputSignals=FCM(4;7)
  Integration : mylib/Integration  SystemSampleTime=-1  VariantActivationTime=update diagram  AllowFlexibleInterface=on  Latency=0  AutoFrameSizeCalculation=off
  YY(4) : Constant  Value=0.4230042431
  "YY(4) " : Outport  VectorParamsAs1DForOutWhenUnconnected=off
  wires:
  CRXR(4)/1 -> Bus Selector/1
  FCM(4,8)/1 -> Bus Selector1/1
  FCM(4,7)/1 -> Bus Selector2/1
  Bus Selector/1 -> " "/3  "<CRXR(4)>"
  Bus Selector1/1 -> " "/2  "<FCM(4;8)>"
  Bus Selector2/1 -> " "/1  "<FCM(4;7)>"
  " "/1 -> Integration/1
  YY(4)/1 -> Integration/2
  Integration/1 -> "YY(4) "/1

== system COSTEP_Auto/Reactor/Holdup of Components in Reactor/YP(5) ==
  FCM(5,7) : Inport
  CRXR(5) : Inport  Port=2
  FCM(5,8) : Inport  Port=3
  " " : Sum  Inputs=+-+
  Bus Selector : BusSelector  OutputSignals=CRXR(5)
  Bus Selector1 : BusSelector  OutputSignals=FCM(5;8)
  Bus Selector2 : BusSelector  OutputSignals=FCM(5;7)
  Integration : mylib/Integration  SystemSampleTime=-1  VariantActivationTime=update diagram  AllowFlexibleInterface=on  Latency=0  AutoFrameSizeCalculation=off
  YY(5) : Constant  Value=24.15513437
  "YY(5) " : Outport  VectorParamsAs1DForOutWhenUnconnected=off
  wires:
  CRXR(5)/1 -> Bus Selector/1
  FCM(5,8)/1 -> Bus Selector1/1
  FCM(5,7)/1 -> Bus Selector2/1
  Bus Selector/1 -> " "/3  "<CRXR(5)>"
  Bus Selector1/1 -> " "/2  "<FCM(5;8)>"
  Bus Selector2/1 -> " "/1  "<FCM(5;7)>"
  " "/1 -> Integration/1
  YY(5)/1 -> Integration/2
  Integration/1 -> "YY(5) "/1

== system COSTEP_Auto/Reactor/Holdup of Components in Reactor/YP(6) ==
  FCM(6,7) : Inport
  CRXR(6) : Inport  Port=2
  FCM(6,8) : Inport  Port=3
  " " : Sum  Inputs=+-+
  Bus Selector : BusSelector  OutputSignals=CRXR(6)
  Bus Selector1 : BusSelector  OutputSignals=FCM(6;8)
  Bus Selector2 : BusSelector  OutputSignals=FCM(6;7)
  Integration : mylib/Integration  SystemSampleTime=-1  VariantActivationTime=update diagram  AllowFlexibleInterface=on  Latency=0  AutoFrameSizeCalculation=off
  YY(6) : Constant  Value=2.942597645
  "YY(6) " : Outport  VectorParamsAs1DForOutWhenUnconnected=off
  wires:
  CRXR(6)/1 -> Bus Selector/1
  FCM(6,8)/1 -> Bus Selector1/1
  FCM(6,7)/1 -> Bus Selector2/1
  Bus Selector/1 -> " "/3  "<CRXR(6)>"
  Bus Selector1/1 -> " "/2  "<FCM(6;8)>"
  Bus Selector2/1 -> " "/1  "<FCM(6;7)>"
  " "/1 -> Integration/1
  YY(6)/1 -> Integration/2
  Integration/1 -> "YY(6) "/1

== system COSTEP_Auto/Reactor/Holdup of Components in Reactor/YP(7) ==
  FCM(7,7) : Inport
  CRXR(7) : Inport  Port=2
  FCM(7,8) : Inport  Port=3
  " " : Sum  Inputs=+-+
  Bus Selector : BusSelector  OutputSignals=CRXR(7)
  Bus Selector1 : BusSelector  OutputSignals=FCM(7;8)
  Bus Selector2 : BusSelector  OutputSignals=FCM(7;7)
  Integration : mylib/Integration  SystemSampleTime=-1  VariantActivationTime=update diagram  AllowFlexibleInterface=on  Latency=0  AutoFrameSizeCalculation=off
  YY(7) : Constant  Value=154.3770655
  "YY(7) " : Outport  VectorParamsAs1DForOutWhenUnconnected=off
  wires:
  CRXR(7)/1 -> Bus Selector/1
  FCM(7,8)/1 -> Bus Selector1/1
  FCM(7,7)/1 -> Bus Selector2/1
  Bus Selector/1 -> " "/3  "<CRXR(7)>"
  Bus Selector1/1 -> " "/2  "<FCM(7;8)>"
  Bus Selector2/1 -> " "/1  "<FCM(7;7)>"
  " "/1 -> Integration/1
  YY(7)/1 -> Integration/2
  Integration/1 -> "YY(7) "/1

== system COSTEP_Auto/Reactor/Holdup of Components in Reactor/YP(8) ==
  FCM(8,7) : Inport
  CRXR(8) : Inport  Port=2
  FCM(8,8) : Inport  Port=3
  " " : Sum  Inputs=+-+
  Bus Selector : BusSelector  OutputSignals=CRXR(8)
  Bus Selector1 : BusSelector  OutputSignals=FCM(8;8)
  Bus Selector2 : BusSelector  OutputSignals=FCM(8;7)
  Integration : mylib/Integration  SystemSampleTime=-1  VariantActivationTime=update diagram  AllowFlexibleInterface=on  Latency=0  AutoFrameSizeCalculation=off
  YY(8) : Constant  Value=159.1865960
  "YY(8) " : Outport  VectorParamsAs1DForOutWhenUnconnected=off
  wires:
  CRXR(8)/1 -> Bus Selector/1
  FCM(8,8)/1 -> Bus Selector1/1
  FCM(8,7)/1 -> Bus Selector2/1
  Bus Selector/1 -> " "/3  "<CRXR(8)>"
  Bus Selector1/1 -> " "/2  "<FCM(8;8)>"
  Bus Selector2/1 -> " "/1  "<FCM(8;7)>"
  " "/1 -> Integration/1
  YY(8)/1 -> Integration/2
  Integration/1 -> "YY(8) "/1
